simulink model "memslab_readout"  (R2019a)
settings: Solver=VariableStepAuto  StartTime=0.0  StopTime=200e-3  MaxStep=1/(2*pi*20e3)/50  RelTol=1e-3
values from neighbouring files (symbols this model uses):
  A_instr = (1+2*Rinstr/Rgain)    (= 9.99992800058)    [memslab_parameters.m]
  A_inv = -R11/R10    (= -2.29166666667)    [memslab_parameters.m]
  CI = 10e-12    (= 1e-11)    [memslab_parameters.m]
  Cs = 5e-12    [memslab_parameters.m]
  dC = 1e-2*Cs    (= 5e-14)    [memslab_parameters.m]
  taulp = Clp*Rlp    (= 0.0024)    [memslab_parameters.m]
settings Model: Creator=dvarx  LastModifiedBy=dvarx

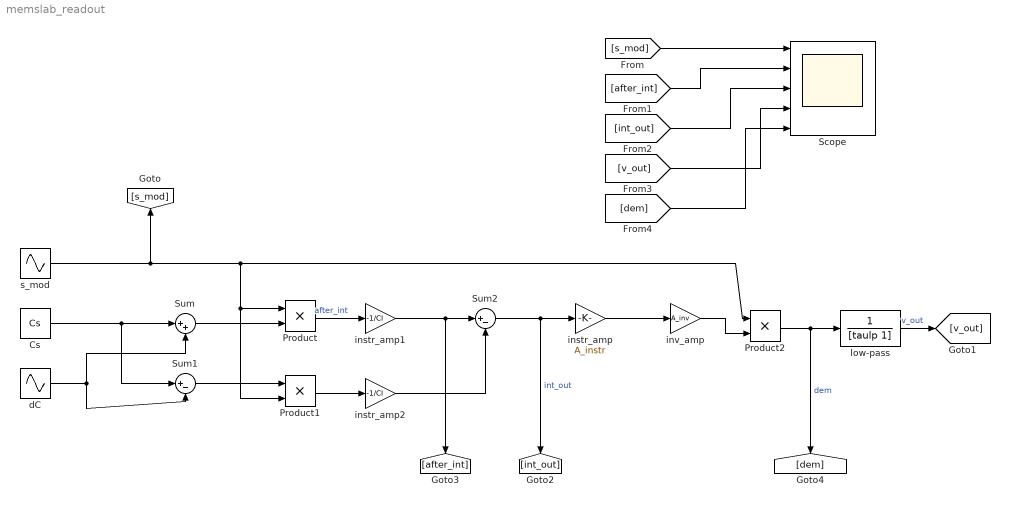
== system memslab_readout ==
  Cs : Constant  Value=Cs
  Product : Product
  Product1 : Product
  Product2 : Product
  Scope : Scope  NumInputPorts=5
  Sum : Sum  Inputs=|++
  Sum1 : Sum  Inputs=|+-
  Sum2 : Sum  Inputs=|+-
  dC : Sin  Amplitude=dC  Frequency=5*2*pi  SampleTime=0
  instr_amp : Gain  Gain=A_instr
  instr_amp1 : Gain  Gain=-1/CI
  instr_amp2 : Gain  Gain=-1/CI
  inv_amp : Gain  Gain=A_inv
  low-pass : TransferFcn  Denominator=[taulp 1]
  s_mod : Sin  Amplitude=5  Frequency=2*pi*20e3  SampleTime=0
  wires:
  Cs/1 -> Sum1/1, Sum/1
  Sum1/1 -> Product1/1
  dC/1 -> Sum1/2, Sum/2
  Product2/1 -> low-pass/1, [dem]  "dem"
  inv_amp/1 -> Product2/2
  low-pass/1 -> [v_out]  "v_out"
  Sum/1 -> Product/2
  instr_amp/1 -> inv_amp/1
  Sum2/1 -> instr_amp/1, [int_out]  "int_out"
  s_mod/1 -> [s_mod], Product/1, Product1/2, Product2/1
  [s_mod] -> Scope/1
  [after_int] -> Scope/2
  [int_out] -> Scope/3
  [v_out] -> Scope/4
  [dem] -> Scope/5
  Product/1 -> instr_amp1/1  "after_int"
  Product1/1 -> instr_amp2/1
  instr_amp1/1 -> [after_int], Sum2/1
  instr_amp2/1 -> Sum2/2
